simulink model "Q3_c_disturbance"  (R2016b)
settings: Solver=VariableStepAuto  StartTime=0.0  StopTime=10.0  RelTol=1e-3
libraries: mpclib x1
settings Model: Creator=Danial  LastModifiedBy=Danial

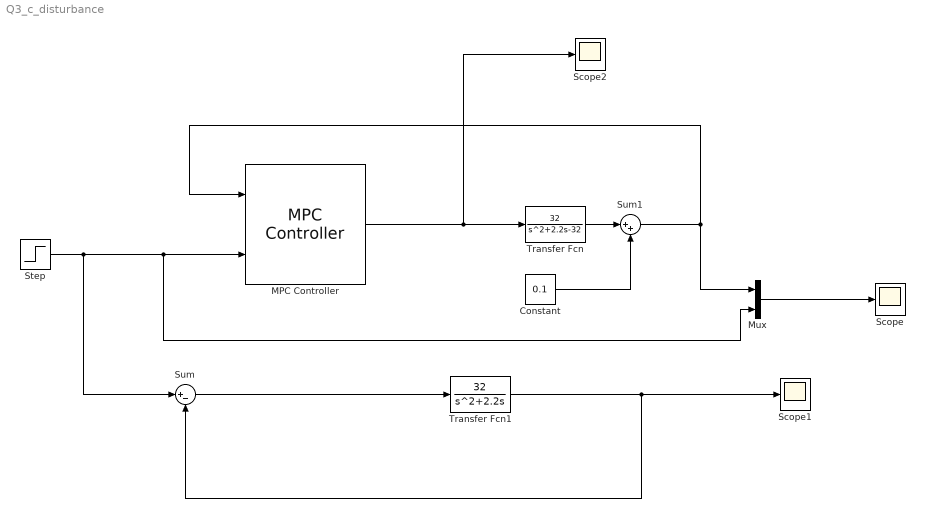
== system Q3_c_disturbance ==
  Constant : Constant  Value=0.1
  MPC Controller : mpclib/MPC Controller  SCDEnableBlockLinearizationSpecification=on  mpcobj=mpcobject  is_multiple=0  enable_value=0  return_u0=off  ref_from_ws=off  ref_signal_name=[]  ref_preview=off  md_from_ws=off  md_signal_name=[]  md_preview=off  from_project=off  project_file=MPCtask.mat  md_inport=off  mv_inport=off  cost_outport=off  return_sequence=off  return_qpstatus=off  return_state=off  state_inport=off  lims_inport=off  ywt_inport=off  is_designfromscratch=0  uwt_inport=off  duwt_inport=off  rhoeps_inport=off  uref_inport=off  n_ts=0.01  n_mv=1  n_md=0  n_ud=0  n_mo=1  n_uo=0  BlockDataType=double  SampleTimeInherited=off  switch_inport=off
  Mux : Mux  Inputs=2
  Scope : Scope
  Scope1 : Scope
  Scope2 : Scope
  Step : Step  SampleTime=0
  Sum : Sum  Inputs=|+-
  Sum1 : Sum  Inputs=|++
  Transfer Fcn : TransferFcn  Numerator=[32]  Denominator=[1 2.2 -32]
  Transfer Fcn1 : TransferFcn  Numerator=[32]  Denominator=[1 2.2 0]
  wires:
  MPC Controller/1 -> Scope2/1, Transfer Fcn/1
  Step/1 -> Sum/1, Mux/2, MPC Controller/2
  Mux/1 -> Scope/1
  Sum/1 -> Transfer Fcn1/1
  Transfer Fcn1/1 -> Scope1/1, Sum/2
  Sum1/1 -> MPC Controller/1, Mux/1
  Transfer Fcn/1 -> Sum1/1
  Constant/1 -> Sum1/2
